simulink model "Testing"  (R2019b)
settings: Solver=VariableStepAuto  StartTime=0.0  StopTime=1000  RelTol=1e-3
values from neighbouring files (symbols this model uses):
  Cdiss = 10E-6    (= 1e-05)    [Model_Run.m]
  Zca = 2    [Model_Run.m]
settings Model: Creator=PranavM  LastModifiedBy=PranavM

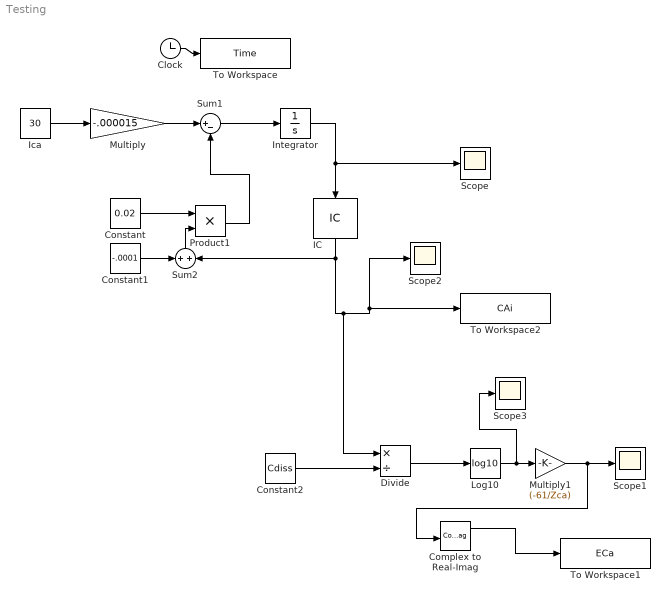
== system Testing ==
  Clock : Clock
  Complex to Real-Imag : ComplexToRealImag
  Constant : Constant  Value=0.02
  Constant1 : Constant  Value=-.0001
  Constant2 : Constant  Value=Cdiss
  Divide : Product  Inputs=*/
  IC : InitialCondition  Value=10E-7
  Ica : Constant  Value=30
  Integrator : Integrator
  Log10 : Math  Operator=log10  SignedPower=off  OutputSignalType=complex  SaturateOnIntegerOverflow=on
  Multiply : Gain  Gain=-.000015
  Multiply1 : Gain  Gain=(-61/Zca)
  Product1 : Product
  Scope{,1..3} (4 alike) : Scope
  Sum1 : Sum  Inputs=|+-
  Sum2 : Sum
  To Workspace : ToWorkspace  VariableName=Time  SampleTime=-1
  To Workspace1 : ToWorkspace  VariableName=ECa  SampleTime=-1
  To Workspace2 : ToWorkspace  VariableName=CAi  SampleTime=-1
  wires:
  Constant1/1 -> Sum2/1
  Ica/1 -> Multiply/1
  Constant/1 -> Product1/1
  Product1/1 -> Sum1/2
  Multiply/1 -> Sum1/1
  IC/1 -> Divide/1, To Workspace2/1, Scope2/1, Sum2/2
  Sum2/1 -> Product1/2
  Sum1/1 -> Integrator/1
  Integrator/1 -> Scope/1, IC/1
  Constant2/1 -> Divide/2
  Divide/1 -> Log10/1
  Log10/1 -> Scope3/1, Multiply1/1
  Multiply1/1 -> Complex to Real-Imag/1, Scope1/1
  Clock/1 -> To Workspace/1
  Complex to Real-Imag/1 -> To Workspace1/1
